simulink model "without_extended_look_ahead"  (R2022a)
settings: Solver=FixedStepAuto  StartTime=0.0  StopTime=18  FixedStep=0.01  RelTol=1e-3
settings Model: Creator=11913  LastModifiedBy=11913

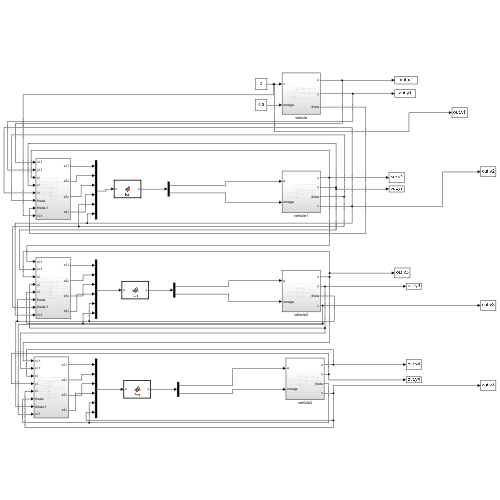
[thumbnail: Simulink's stored preview of the top-level diagram]
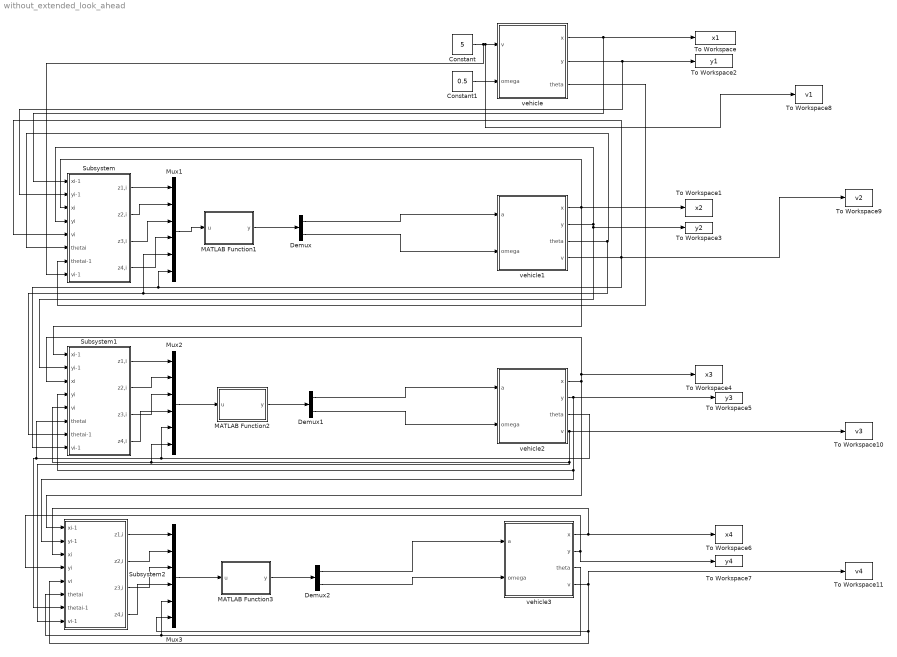
== system without_extended_look_ahead ==
  Constant : Constant  Value=5
  Constant1 : Constant  Value=0.5
  Demux : Demux  Outputs=2
  Demux1 : Demux  Outputs=2
  Demux2 : Demux  Outputs=2
  MATLAB Function1 : MATLAB Function  TreatAsAtomicUnit=on
  MATLAB Function2 : MATLAB Function  TreatAsAtomicUnit=on
  MATLAB Function3 : MATLAB Function  TreatAsAtomicUnit=on
  Mux1 : Mux  Inputs=6
  Mux2 : Mux  Inputs=6
  Mux3 : Mux  Inputs=6
  Subsystem : Subsystem
  Subsystem1 : Subsystem
  Subsystem2 : Subsystem
  To Workspace : ToWorkspace  VariableName=x1  SampleTime=-1
      settings: Save2DSignal=2-D array (concatenate along first dimension)
  To Workspace1 : ToWorkspace  VariableName=x2  SampleTime=-1
      settings: Save2DSignal=2-D array (concatenate along first dimension)
  To Workspace10 : ToWorkspace  VariableName=v3  SaveFormat=Timeseries  SampleTime=-1
      settings: Save2DSignal=2-D array (concatenate along first dimension)
  To Workspace11 : ToWorkspace  VariableName=v4  SaveFormat=Timeseries  SampleTime=-1
      settings: Save2DSignal=2-D array (concatenate along first dimension)
  To Workspace2 : ToWorkspace  VariableName=y1  SampleTime=-1
      settings: Save2DSignal=2-D array (concatenate along first dimension)
  To Workspace3 : ToWorkspace  VariableName=y2  SampleTime=-1
      settings: Save2DSignal=2-D array (concatenate along first dimension)
  To Workspace4 : ToWorkspace  VariableName=x3  SampleTime=-1
      settings: Save2DSignal=2-D array (concatenate along first dimension)
  To Workspace5 : ToWorkspace  VariableName=y3  SampleTime=-1
      settings: Save2DSignal=2-D array (concatenate along first dimension)
  To Workspace6 : ToWorkspace  VariableName=x4  SampleTime=-1
      settings: Save2DSignal=2-D array (concatenate along first dimension)
  To Workspace7 : ToWorkspace  VariableName=y4  SampleTime=-1
      settings: Save2DSignal=2-D array (concatenate along first dimension)
  To Workspace8 : ToWorkspace  VariableName=v1  SaveFormat=Timeseries  SampleTime=-1
      settings: Save2DSignal=2-D array (concatenate along first dimension)
  To Workspace9 : ToWorkspace  VariableName=v2  SaveFormat=Timeseries  SampleTime=-1
      settings: Save2DSignal=2-D array (concatenate along first dimension)
  vehicle : Subsystem
  vehicle1 : Subsystem
  vehicle2 : Subsystem
  vehicle3 : Subsystem
  wires:
  Constant/1 -> Subsystem/8(vi-1), To Workspace8/1, vehicle/1(v)
  Constant1/1 -> vehicle/2(omega)
  vehicle/2(y) -> To Workspace2/1, Subsystem/2(yi-1)
  vehicle/1(x) -> To Workspace/1, Subsystem/1(xi-1)
  vehicle/3(theta) -> Subsystem/7(thetai-1)
  vehicle1/1(x) -> Subsystem1/1(xi-1), To Workspace1/1, Subsystem/3(xi)
  vehicle1/2(y) -> Subsystem1/2(yi-1), To Workspace3/1, Subsystem/4(yi)
  vehicle1/4(v) -> Subsystem/5(vi), To Workspace9/1, Subsystem1/8(vi-1), Mux1/6
  vehicle1/3(theta) -> Subsystem1/7(thetai-1), Mux1/5, Subsystem/6(thetai)
  Subsystem/1(z1,i) -> Mux1/1
  Subsystem/2(z2,i) -> Mux1/2
  Subsystem/3(z3,i) -> Mux1/3
  Subsystem/4(z4,i) -> Mux1/4
  Mux1/1 -> MATLAB Function1/1(u)
  Demux/1 -> vehicle1/1(a)
  Demux/2 -> vehicle1/2(omega)
  MATLAB Function1/1(y) -> Demux/1
  vehicle2/1(x) -> To Workspace4/1, Subsystem1/3(xi), Subsystem2/1(xi-1)
  vehicle2/2(y) -> Subsystem2/2(yi-1), Subsystem1/4(yi), To Workspace5/1
  vehicle2/4(v) -> To Workspace10/1, Subsystem2/8(vi-1), Mux2/6, Subsystem1/5(vi)
  vehicle2/3(theta) -> Subsystem2/7(thetai-1), Subsystem1/6(thetai), Mux2/5
  Subsystem1/1(z1,i) -> Mux2/1
  Subsystem1/2(z2,i) -> Mux2/2
  Subsystem1/3(z3,i) -> Mux2/3
  Subsystem1/4(z4,i) -> Mux2/4
  Mux2/1 -> MATLAB Function2/1(u)
  MATLAB Function2/1(y) -> Demux1/1
  Demux1/1 -> vehicle2/1(a)
  Demux1/2 -> vehicle2/2(omega)
  vehicle3/1(x) -> To Workspace6/1, Subsystem2/3(xi)
  vehicle3/2(y) -> To Workspace7/1, Subsystem2/4(yi)
  vehicle3/4(v) -> Mux3/6, Subsystem2/5(vi), To Workspace11/1
  vehicle3/3(theta) -> Mux3/5, Subsystem2/6(thetai)
  Subsystem2/1(z1,i) -> Mux3/1
  Subsystem2/2(z2,i) -> Mux3/2
  Subsystem2/3(z3,i) -> Mux3/3
  Subsystem2/4(z4,i) -> Mux3/4
  Mux3/1 -> MATLAB Function3/1(u)
  MATLAB Function3/1(y) -> Demux2/1
  Demux2/1 -> vehicle3/1(a)
  Demux2/2 -> vehicle3/2(omega)

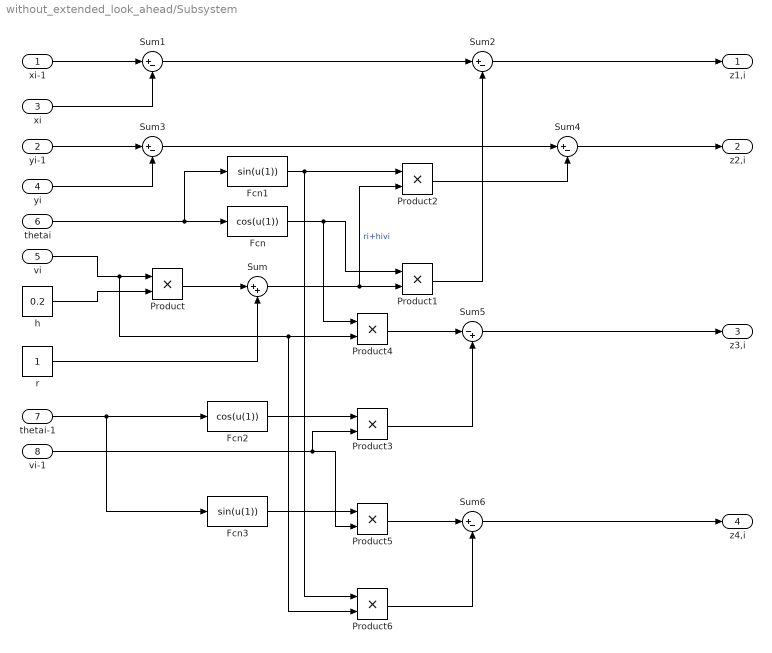
== system without_extended_look_ahead/Subsystem ==
  xi-1 : Inport
  yi-1 : Inport  Port=2
  xi : Inport  Port=3
  yi : Inport  Port=4
  vi : Inport  Port=5
  thetai : Inport  Port=6
  thetai-1 : Inport  Port=7
  vi-1 : Inport  Port=8
  Fcn : Fcn  Expr=cos(u(1))
  Fcn1 : Fcn  Expr=sin(u(1))
  Fcn2 : Fcn  Expr=cos(u(1))
  Fcn3 : Fcn  Expr=sin(u(1))
  Product{,1..6} (7 alike) : Product
  Sum : Sum  Inputs=|++
  Sum{1..4,6} (5 alike) : Sum  Inputs=|+-
  Sum5 : Sum  Inputs=|-+
  h : Constant  Value=0.2
  r : Constant
  z1,i : Outport
  z2,i : Outport  Port=2
  z3,i : Outport  Port=3
  z4,i : Outport  Port=4
  wires:
  vi/1 -> Product6/2, Product4/2, Product/1
  h/1 -> Product/2
  Product/1 -> Sum/1
  r/1 -> Sum/2
  xi-1/1 -> Sum1/1
  xi/1 -> Sum1/2
  thetai/1 -> Fcn1/1, Fcn/1
  Sum/1 -> Product2/2, Product1/2  "ri+hivi"
  Fcn/1 -> Product4/1, Product1/1
  Sum1/1 -> Sum2/1
  Product1/1 -> Sum2/2
  yi-1/1 -> Sum3/1
  yi/1 -> Sum3/2
  Fcn1/1 -> Product6/1, Product2/1
  Sum3/1 -> Sum4/1
  Product2/1 -> Sum4/2
  Sum4/1 -> z2,i/1
  Sum2/1 -> z1,i/1
  thetai-1/1 -> Fcn3/1, Fcn2/1
  Fcn2/1 -> Product3/1
  vi-1/1 -> Product5/2, Product3/2
  Product3/1 -> Sum5/2
  Product4/1 -> Sum5/1
  Sum5/1 -> z3,i/1
  Fcn3/1 -> Product5/1
  Product5/1 -> Sum6/1
  Product6/1 -> Sum6/2
  Sum6/1 -> z4,i/1

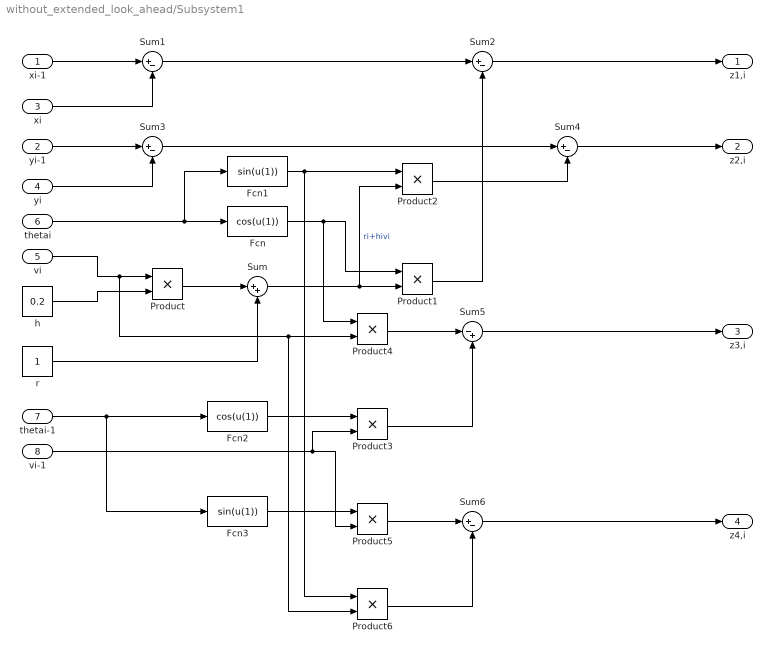
== system without_extended_look_ahead/Subsystem1 ==
  xi-1 : Inport
  yi-1 : Inport  Port=2
  xi : Inport  Port=3
  yi : Inport  Port=4
  vi : Inport  Port=5
  thetai : Inport  Port=6
  thetai-1 : Inport  Port=7
  vi-1 : Inport  Port=8
  Fcn : Fcn  Expr=cos(u(1))
  Fcn1 : Fcn  Expr=sin(u(1))
  Fcn2 : Fcn  Expr=cos(u(1))
  Fcn3 : Fcn  Expr=sin(u(1))
  Product{,1..6} (7 alike) : Product
  Sum : Sum  Inputs=|++
  Sum{1..4,6} (5 alike) : Sum  Inputs=|+-
  Sum5 : Sum  Inputs=|-+
  h : Constant  Value=0.2
  r : Constant
  z1,i : Outport
  z2,i : Outport  Port=2
  z3,i : Outport  Port=3
  z4,i : Outport  Port=4
  wires:
  vi/1 -> Product6/2, Product4/2, Product/1
  h/1 -> Product/2
  Product/1 -> Sum/1
  r/1 -> Sum/2
  xi-1/1 -> Sum1/1
  xi/1 -> Sum1/2
  thetai/1 -> Fcn1/1, Fcn/1
  Sum/1 -> Product2/2, Product1/2  "ri+hivi"
  Fcn/1 -> Product4/1, Product1/1
  Sum1/1 -> Sum2/1
  Product1/1 -> Sum2/2
  yi-1/1 -> Sum3/1
  yi/1 -> Sum3/2
  Fcn1/1 -> Product6/1, Product2/1
  Sum3/1 -> Sum4/1
  Product2/1 -> Sum4/2
  Sum4/1 -> z2,i/1
  Sum2/1 -> z1,i/1
  thetai-1/1 -> Fcn3/1, Fcn2/1
  Fcn2/1 -> Product3/1
  vi-1/1 -> Product5/2, Product3/2
  Product3/1 -> Sum5/2
  Product4/1 -> Sum5/1
  Sum5/1 -> z3,i/1
  Fcn3/1 -> Product5/1
  Product5/1 -> Sum6/1
  Product6/1 -> Sum6/2
  Sum6/1 -> z4,i/1

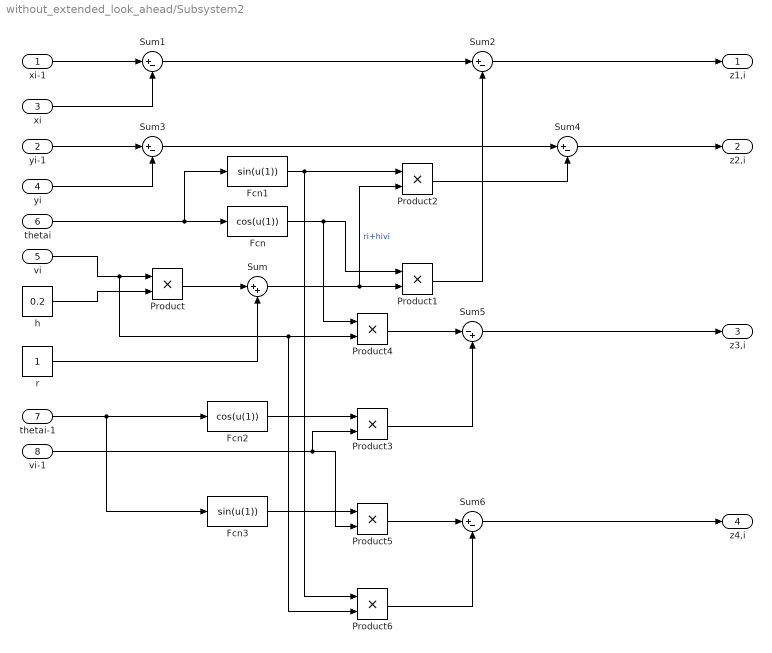
== system without_extended_look_ahead/Subsystem2 ==
  xi-1 : Inport
  yi-1 : Inport  Port=2
  xi : Inport  Port=3
  yi : Inport  Port=4
  vi : Inport  Port=5
  thetai : Inport  Port=6
  thetai-1 : Inport  Port=7
  vi-1 : Inport  Port=8
  Fcn : Fcn  Expr=cos(u(1))
  Fcn1 : Fcn  Expr=sin(u(1))
  Fcn2 : Fcn  Expr=cos(u(1))
  Fcn3 : Fcn  Expr=sin(u(1))
  Product{,1..6} (7 alike) : Product
  Sum : Sum  Inputs=|++
  Sum{1..4,6} (5 alike) : Sum  Inputs=|+-
  Sum5 : Sum  Inputs=|-+
  h : Constant  Value=0.2
  r : Constant
  z1,i : Outport
  z2,i : Outport  Port=2
  z3,i : Outport  Port=3
  z4,i : Outport  Port=4
  wires:
  vi/1 -> Product6/2, Product4/2, Product/1
  h/1 -> Product/2
  Product/1 -> Sum/1
  r/1 -> Sum/2
  xi-1/1 -> Sum1/1
  xi/1 -> Sum1/2
  thetai/1 -> Fcn1/1, Fcn/1
  Sum/1 -> Product2/2, Product1/2  "ri+hivi"
  Fcn/1 -> Product4/1, Product1/1
  Sum1/1 -> Sum2/1
  Product1/1 -> Sum2/2
  yi-1/1 -> Sum3/1
  yi/1 -> Sum3/2
  Fcn1/1 -> Product6/1, Product2/1
  Sum3/1 -> Sum4/1
  Product2/1 -> Sum4/2
  Sum4/1 -> z2,i/1
  Sum2/1 -> z1,i/1
  thetai-1/1 -> Fcn3/1, Fcn2/1
  Fcn2/1 -> Product3/1
  vi-1/1 -> Product5/2, Product3/2
  Product3/1 -> Sum5/2
  Product4/1 -> Sum5/1
  Sum5/1 -> z3,i/1
  Fcn3/1 -> Product5/1
  Product5/1 -> Sum6/1
  Product6/1 -> Sum6/2
  Sum6/1 -> z4,i/1

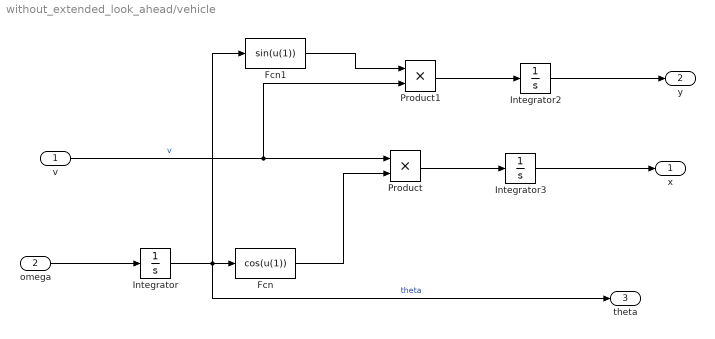
== system without_extended_look_ahead/vehicle ==
  v : Inport
  omega : Inport  Port=2
  Fcn : Fcn  Expr=cos(u(1))
  Fcn1 : Fcn  Expr=sin(u(1))
  Integrator : Integrator
  Integrator2 : Integrator
  Integrator3 : Integrator
  Product : Product
  Product1 : Product
  x : Outport
  y : Outport  Port=2
  theta : Outport  Port=3
  wires:
  omega/1 -> Integrator/1
  Integrator/1 -> theta/1, Fcn1/1, Fcn/1  "theta"
  v/1 -> Product1/2, Product/1  "v"
  Fcn/1 -> Product/2
  Fcn1/1 -> Product1/1
  Product1/1 -> Integrator2/1
  Product/1 -> Integrator3/1
  Integrator2/1 -> y/1
  Integrator3/1 -> x/1

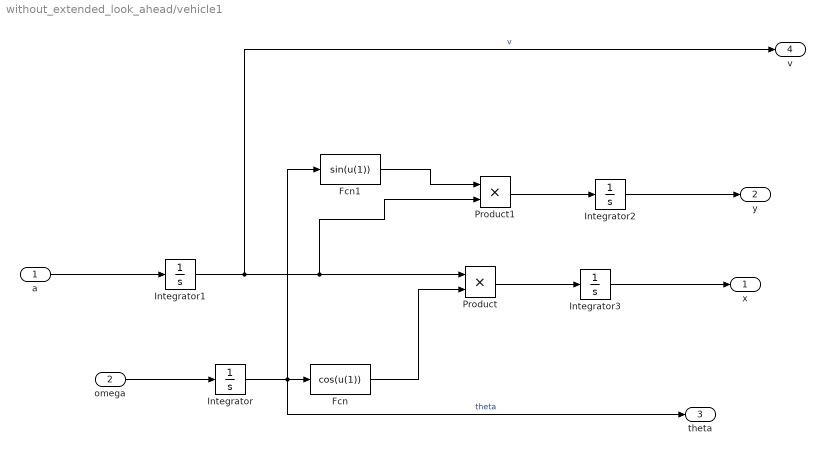
== system without_extended_look_ahead/vehicle1 ==
  a : Inport
  omega : Inport  Port=2
  Fcn : Fcn  Expr=cos(u(1))
  Fcn1 : Fcn  Expr=sin(u(1))
  Integrator : Integrator
  Integrator1 : Integrator  InitialCondition=5
  Integrator2 : Integrator  InitialCondition=2
  Integrator3 : Integrator  InitialCondition=-2
  Product : Product
  Product1 : Product
  x : Outport
  y : Outport  Port=2
  theta : Outport  Port=3
  v : Outport  Port=4
  wires:
  omega/1 -> Integrator/1
  Integrator/1 -> theta/1, Fcn1/1, Fcn/1  "theta"
  Fcn/1 -> Product/2
  Fcn1/1 -> Product1/1
  Product1/1 -> Integrator2/1
  Product/1 -> Integrator3/1
  Integrator2/1 -> y/1
  Integrator3/1 -> x/1
  a/1 -> Integrator1/1
  Integrator1/1 -> v/1, Product1/2, Product/1  "v"

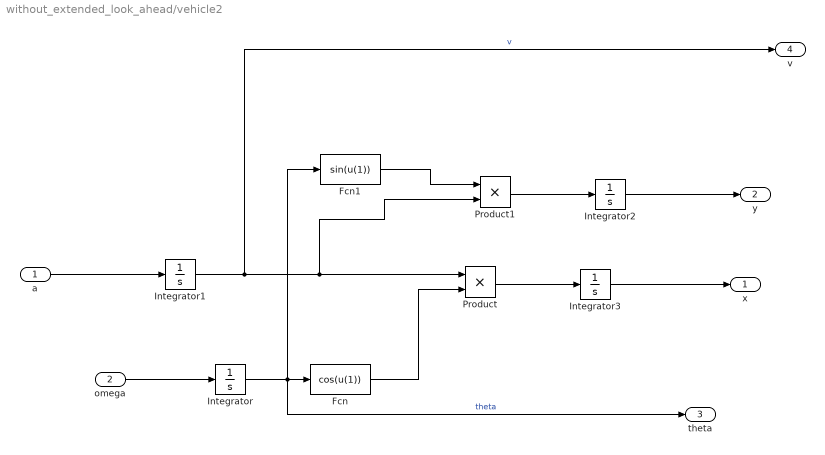
== system without_extended_look_ahead/vehicle2 ==
  a : Inport
  omega : Inport  Port=2
  Fcn : Fcn  Expr=cos(u(1))
  Fcn1 : Fcn  Expr=sin(u(1))
  Integrator : Integrator
  Integrator1 : Integrator  InitialCondition=5
  Integrator2 : Integrator  InitialCondition=4
  Integrator3 : Integrator  InitialCondition=-4
  Product : Product
  Product1 : Product
  x : Outport
  y : Outport  Port=2
  theta : Outport  Port=3
  v : Outport  Port=4
  wires:
  omega/1 -> Integrator/1
  Integrator/1 -> theta/1, Fcn1/1, Fcn/1  "theta"
  Fcn/1 -> Product/2
  Fcn1/1 -> Product1/1
  Product1/1 -> Integrator2/1
  Product/1 -> Integrator3/1
  Integrator2/1 -> y/1
  Integrator3/1 -> x/1
  a/1 -> Integrator1/1
  Integrator1/1 -> v/1, Product1/2, Product/1  "v"

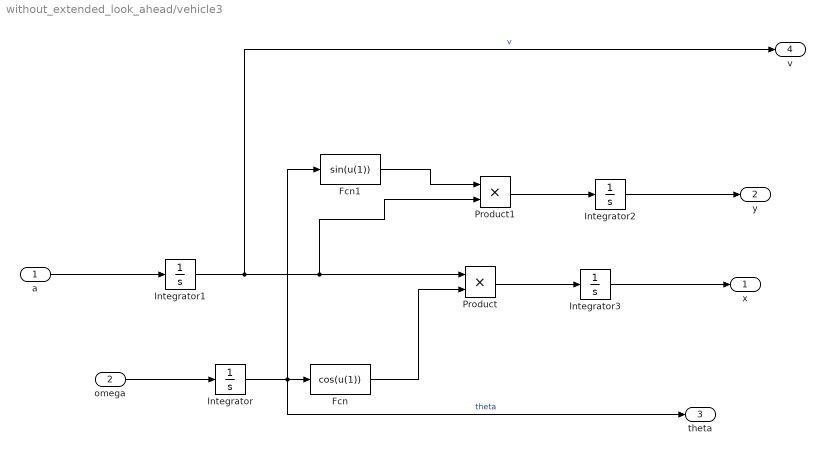
== system without_extended_look_ahead/vehicle3 ==
  a : Inport
  omega : Inport  Port=2
  Fcn : Fcn  Expr=cos(u(1))
  Fcn1 : Fcn  Expr=sin(u(1))
  Integrator : Integrator
  Integrator1 : Integrator  InitialCondition=5
  Integrator2 : Integrator  InitialCondition=6
  Integrator3 : Integrator  InitialCondition=-6
  Product : Product
  Product1 : Product
  x : Outport
  y : Outport  Port=2
  theta : Outport  Port=3
  v : Outport  Port=4
  wires:
  omega/1 -> Integrator/1
  Integrator/1 -> theta/1, Fcn1/1, Fcn/1  "theta"
  Fcn/1 -> Product/2
  Fcn1/1 -> Product1/1
  Product1/1 -> Integrator2/1
  Product/1 -> Integrator3/1
  Integrator2/1 -> y/1
  Integrator3/1 -> x/1
  a/1 -> Integrator1/1
  Integrator1/1 -> v/1, Product1/2, Product/1  "v"

== matlab function without_extended_look_ahead/MATLAB Function2 ==
  data: u input; y output
function y = fcn(u)
z1_i=u(1);
z2_i=u(2);
z3_i=u(3);
z4_i=u(4);
thetai=u(5);
vi=u(6);

k1=3.5;
k2=3.5;
u1=z3_i+k1*z1_i;
u2=z4_i+k2*z2_i;
r=1;
h=0.2;

F11=h*cos(thetai);
F12=-(r+h*vi)*sin(thetai);
F21=h*sin(thetai);
F22=(r+h*vi)*cos(thetai);
F = [F11,F12;F21,F22];

F_inv = F \ eye(2);%计算F的逆矩阵

y = F_inv*[u1;u2];

== matlab function without_extended_look_ahead/MATLAB Function3 ==
  data: u input; y output
function y = fcn(u)
z1_i=u(1);
z2_i=u(2);
z3_i=u(3);
z4_i=u(4);
thetai=u(5);
vi=u(6);

k1=3.5;
k2=3.5;
u1=z3_i+k1*z1_i;
u2=z4_i+k2*z2_i;
r=1;
h=0.2;

F11=h*cos(thetai);
F12=-(r+h*vi)*sin(thetai);
F21=h*sin(thetai);
F22=(r+h*vi)*cos(thetai);
F = [F11,F12;F21,F22];

F_inv = F \ eye(2);%计算F的逆矩阵

y = F_inv*[u1;u2];

== matlab function without_extended_look_ahead/MATLAB Function1 ==
  data: u input; y output
function y = fcn(u)
z1_i=u(1);
z2_i=u(2);
z3_i=u(3);
z4_i=u(4);
thetai=u(5);
vi=u(6);

k1=3.5;
k2=3.5;
u1=z3_i+k1*z1_i;
u2=z4_i+k2*z2_i;
r=1;
h=0.2;

F11=h*cos(thetai);
F12=-(r+h*vi)*sin(thetai);
F21=h*sin(thetai);
F22=(r+h*vi)*cos(thetai);
F = [F11,F12;F21,F22];

F_inv = F \ eye(2);%计算F的逆矩阵

y = F_inv*[u1;u2];
